simulink model "untitled"  (R2024b)
settings: Solver=VariableStepAuto  StartTime=0.0  StopTime=10.0  RelTol=1e-3
settings Model: Creator=christopherwaight  LastModifiedBy=christopherwaight

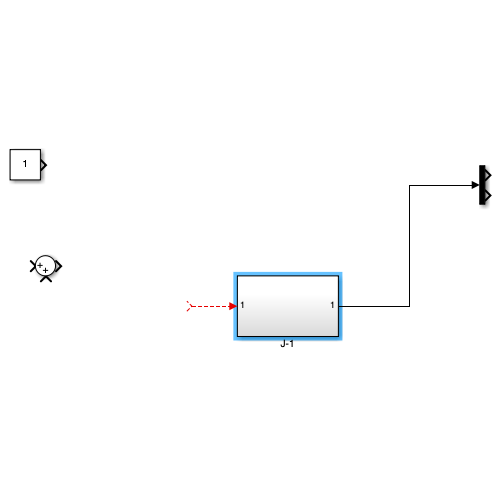
[thumbnail: Simulink's stored preview of the top-level diagram]
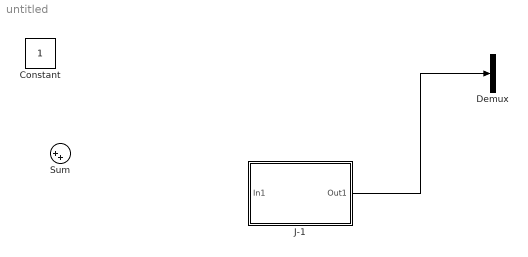
== system untitled ==
  Constant : Constant
  Demux : Demux  Outputs=2
  J-1 : Subsystem
  Sum : Sum  Inputs=|++
  wires:
  ? -> J-1/1(In1)
  J-1/1(Out1) -> Demux/1

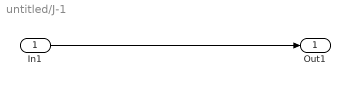
== system untitled/J-1 ==
  In1 : Inport
  Out1 : Outport
  wires:
  In1/1 -> Out1/1
